simulink model "NonlinearModel_LinearController"  (R2017b)
settings: Solver=ode4  StartTime=0.0  StopTime=time  FixedStep=step_size  RelTol=1e-3
values from neighbouring files (symbols this model uses):
  K = acker(A,B,pc)    [FeedbackGain.m]    (also in LinearisedModel.m = acker(A_,B,pc); integral_control.m; matlab.mat = 0; nat_freq_stable_sys.m = -f2)
  motor_stall_torque = 8    [LinearAnimations.m]    (also in LinearisedModel.m = 2.8; NonLinearAnimations.m; experiment_vs_simulated.m)
  phi_dot_start = 0    [LinearAnimations.m]    (also in NonLinearAnimations.m = -0.5; experiment_vs_simulated.m)
  phi_start = 0    [LinearAnimations.m]    (also in NonLinearAnimations.m; experiment_vs_simulated.m = -1.502)
  theta_dot_start = 0    [LinearAnimations.m]    (also in NonLinearAnimations.m; experiment_vs_simulated.m)
  theta_start = pi + pi/100    (= 3.17300858013)    [LinearAnimations.m]    (also in NonLinearAnimations.m = 0; experiment_vs_simulated.m = 0)
settings Model: Creator=Henry  LastModifiedBy=Henry
settings CodeAppCC: StateflowObjectComments=on

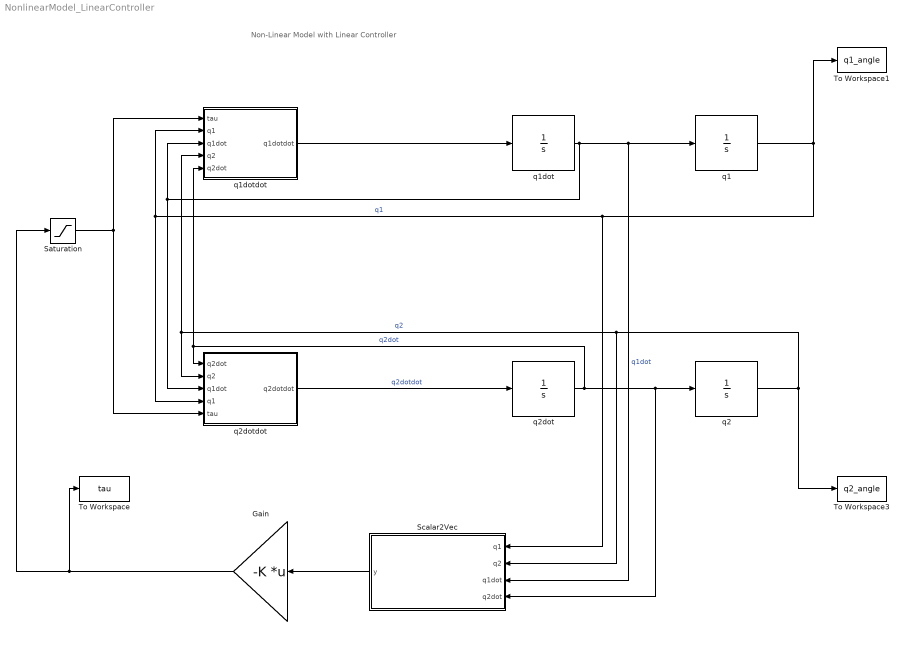
== system NonlinearModel_LinearController ==
  note: Non-Linear Model with Linear Controller
  Gain : Gain  Gain=-K  Multiplication=Matrix(K*u)
  Saturation : Saturate  UpperLimit=motor_stall_torque  LowerLimit=-1*motor_stall_torque
  Scalar2Vec : MATLAB Function  TreatAsAtomicUnit=on
  To Workspace : ToWorkspace  VariableName=tau  SaveFormat=Timeseries  SampleTime=-1
  To Workspace1 : ToWorkspace  VariableName=q1_angle  SaveFormat=Timeseries  SampleTime=-1
  To Workspace3 : ToWorkspace  VariableName=q2_angle  SaveFormat=Timeseries  SampleTime=-1
  q1 : Integrator  InitialCondition=theta_start  ContinuousStateAttributes='angle_q1'
  q1dot : Integrator  InitialCondition=theta_dot_start
  q1dotdot : MATLAB Function  TreatAsAtomicUnit=on
  q2 : Integrator  InitialCondition=phi_start  ContinuousStateAttributes='angle_2'
  q2dot : Integrator  InitialCondition=phi_dot_start
  q2dotdot : MATLAB Function  TreatAsAtomicUnit=on
  wires:
  Gain/1 -> To Workspace/1, Saturation/1
  q1/1 -> Scalar2Vec/1(q1), q2dotdot/4(q1), q1dotdot/2(q1), To Workspace1/1  "q1"
  q2/1 -> To Workspace3/1, Scalar2Vec/2(q2), q1dotdot/4(q2), q2dotdot/2(q2)  "q2"
  q2dot/1 -> q2dotdot/1(q2dot), q1dotdot/5(q2dot), Scalar2Vec/4(q2dot), q2/1  "q2dot"
  q2dotdot/1(q2dotdot) -> q2dot/1  "q2dotdot"
  q1dotdot/1(q1dotdot) -> q1dot/1
  q1dot/1 -> q2dotdot/3(q1dot), q1dotdot/3(q1dot), Scalar2Vec/3(q1dot), q1/1  "q1dot"
  Scalar2Vec/1(y) -> Gain/1
  Saturation/1 -> q2dotdot/5(tau), q1dotdot/1(tau)

== matlab function NonlinearModel_LinearController/q2dotdot ==
  data: q2dot input; q2 input; q1dot input; q1 input; tau input; q2dotdot output
function q2dotdot = fcn(q2dot, q2, q1dot,q1, tau)

%% System Constants
g = 9.81;
Ia = 0.0265152541;
Ib = 0.0221429705;
L1 = 0.2350;
L2 = 0.245;
l1 = 0.235;
l2 = 0.2450;
m1 = 0.5763;
m2 = 0.49277;
f1 = 0;
f2 = 0;

%% System Dynamics
A = Ia+Ib+m2*L1^2+m2*l2^2+2*m2*l2*L1*cos(q2);
B = Ib+m2*l2^2+m2*L1*l2*cos(q2);
E = m1*g*l1*sin(q1);
F = m2*g*L1*sin(q1);
G = m2*g*l2*sin(q1+q2);
C = 2*m2*l2*L1*q1dot*q2dot*sin(q2);
D = m2*L1*l2*q2dot^2*sin(q2);

H =Ib+m2*l2^2+m2*L1*l2*cos(q2);
I =Ib+m2*l2^2;
K = m2*L1*l2*q1dot^2*sin(q2);
J = m2*L1*l2*q1dot*q2dot*sin(q2);
M = m2*g*l2*sin(q1+q2);
L = m2*L1*l2*q1dot*q2dot*sin(q2);
% Coefficient for Damping 

Z = -f1*q1dot;
Y = -f2*(q2dot-q1dot)+tau;

alpha = -C-D+E+F+G-Z;
zeta = -J+K+L+M-Y;

AA = [A,B;H,I];
BB = [-alpha;-zeta];

meep = AA\BB;
q2dotdot = meep(end,1);

== matlab function NonlinearModel_LinearController/q1dotdot ==
  data: tau input; q1 input; q1dot input; q2 input; q2dot input; q1dotdot output
function q1dotdot = fcn(tau, q1, q1dot,q2, q2dot)

%% System Constants
g = 9.81;
Ia = 0.0265152541;
Ib = 0.0221429705;
L1 = 0.2350;
L2 = 0.245;
l1 = 0.235;
l2 =  0.2450;
m1 = 0.5763;
m2 = 0.49277;
f1 = 0;
f2 = 0;

%% System Dynamics
A = Ia+Ib+m2*L1^2+m2*l2^2+2*m2*l2*L1*cos(q2);
B = Ib+m2*l2^2+m2*L1*l2*cos(q2);
E = m1*g*l1*sin(q1);
F = m2*g*L1*sin(q1);
G = m2*g*l2*sin(q1+q2);
C = 2*m2*l2*L1*q1dot*q2dot*sin(q2);
D = m2*L1*l2*q2dot^2*sin(q2);

H = Ib+m2*l2^2+m2*L1*l2*cos(q2);
I = Ib+m2*l2^2;
K = m2*L1*l2*q1dot^2*sin(q2);
J = m2*L1*l2*q1dot*q2dot*sin(q2);
M = m2*g*l2*sin(q1+q2);
L = m2*L1*l2*q1dot*q2dot*sin(q2);
% Coefficient for Damping 
Z = -f1*q1dot;
Y = -f2*(q2dot-q1dot)+tau;

alpha = -C-D+E+F+G-Z;
zeta = -J+K+L+M-Y;

AA = [A,B;H,I];
BB = [-alpha;-zeta];

meep = AA\BB;
q1dotdot = meep(1,1);

== matlab function NonlinearModel_LinearController/Scalar2Vec ==
  data: q1 input; y output; q2 input; q1dot input; q2dot input
function y = fcn(q1,q2,q1dot,q2dot)

y = [q1-pi;q2;q1dot;q2dot];
